simulink model "PID0"  (R2020b)
settings: Solver=VariableStepAuto  StartTime=0.0  StopTime=1  RelTol=1e-3
model workspace (MAT data in the model file):
  Kd = Simulink.Parameter
  Kd.Value = 49.1069
  Kd.DataType = 'auto'
  Kd.Dimensions = [1 1]
  Ki = Simulink.Parameter
  Ki.Value = 3902603746
  Ki.DataType = 'auto'
  Ki.Dimensions = [1 1]
  Kp = Simulink.Parameter
  Kp.Value = 881695.95
  Kp.DataType = 'auto'
  Kp.Dimensions = [1 1]
values from neighbouring files (symbols this model uses):
  Kd = 49.1069    [data.sldd]
  Ki = 3902603745.9987    [data.sldd]
  Kp = 881695.95    [data.sldd]
settings Model: DataDictionary=data.sldd  Creator=smart  LastModifiedBy=smart
settings DataIOCC: SaveOutput=off  SaveTime=off

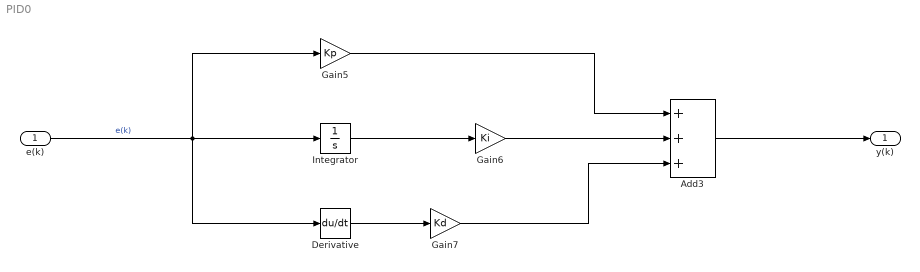
== system PID0 ==
  e(k) : Inport  OutDataTypeStr=double  PortDimensions=1  SampleTime=0
  Add3 : Sum  Inputs=+++
  Derivative : Derivative
  Gain5 : Gain  Gain=Kp
  Gain6 : Gain  Gain=Ki
  Gain7 : Gain  Gain=Kd
  Integrator : Integrator
  y(k) : Outport  OutDataTypeStr=double  PortDimensions=1  SampleTime=0
  wires:
  Gain6/1 -> Add3/2
  Add3/1 -> y(k)/1
  Derivative/1 -> Gain7/1
  Integrator/1 -> Gain6/1
  e(k)/1 -> Gain5/1, Integrator/1, Derivative/1  "e(k)"
  Gain5/1 -> Add3/1
  Gain7/1 -> Add3/3
